simulink model "mrefrobotarm_modified_previous_y_previous_u_previous_ref"  (R2018b)
settings: Solver=FixedStepAuto  StartTime=0.0  StopTime=10  RelTol=1e-3  AbsTol=1e-6
undefined symbols (not defined in the file or in its folder): options, sfunxy2
libraries: neural x949, simulink x1
(part 16 of 31)

== system mrefrobotarm_modified_previous_y_previous_u_previous_ref/const_51_unstable/Layer 2/Delays 1 ==
  "p{2}" : Inport  PortDimensions=50
      mask Display: e = 0.06;c1 = [120 230 180]/255;c2 = ([120 230 180]+0)/(256+128);c3 = ([120 230 180]+128)/(256+128);patch([0 1 1 0],[0 0 1 1],c1);patch([0 1 1 1-e 1-e 0+e],[0 0 1 1-e 0+e 0+e],c2);patch([0 0 1 1-e 0+e 0+e],[0 1 1 1-e 1-e 0+e],c3);plot([0 1 1 0 0],[0 0 1 1 0]);
  mux : Mux  Inputs=1
      mask Display: e = 0.06;c1 = [120 150 230]/255;c2 = ([120 150 230]+0)/383;c3 = ([120 150 230]+128)/383;patch([0 1 1 0],[0 0 1 1],c1);patch([0 1 1 1-e 1-e 0+e],[0 0 1 1-e 0+e 0+e],c2);patch([0 0 1 1-e 0+e 0+e],[0 1 1 1-e 1-e 0+e],c3);plot([0 1 1 0 0],[0 0 1 1 0]);disp('Mux')
  "pd{2,1}" : Outport
      mask Display: e = 0.06;c1 = [120 230 180]/255;c2 = ([120 230 180]+0)/(256+128);c3 = ([120 230 180]+128)/(256+128);patch([0 1 1 0],[0 0 1 1],c1);patch([0 1 1 1-e 1-e 0+e],[0 0 1 1-e 0+e 0+e],c2);patch([0 0 1 1-e 0+e 0+e],[0 1 1 1-e 1-e 0+e],c3);plot([0 1 1 0 0],[0 0 1 1 0]);
  wires:
  "p{2}"/1 -> mux/1
  mux/1 -> "pd{2,1}"/1

== system mrefrobotarm_modified_previous_y_previous_u_previous_ref/const_51_unstable/Layer 2/LW{2,1} ==
  "ad{2,1}" : Inport  PortDimensions=50
      mask Display: e = 0.06;c1 = [120 230 180]/255;c2 = ([120 230 180]+0)/(256+128);c3 = ([120 230 180]+128)/(256+128);patch([0 1 1 0],[0 0 1 1],c1);patch([0 1 1 1-e 1-e 0+e],[0 0 1 1-e 0+e 0+e],c2);patch([0 0 1 1-e 0+e 0+e],[0 1 1 1-e 1-e 0+e],c3);plot([0 1 1 0 0],[0 0 1 1 0]);
  "IW{2,1}(1,:)'" : Constant  Value=[0.015906593054590668911973949661842198111116886138916015625;0.01820805169246907107005739590022130869328975677490234375;0.326514062945760741296652440723846666514873504638671875;-0.1966668405829790078342966808122582733631134033203125;0.50794780405529216249504997904296033084392547607421875;-1.7723192755342032089771464598015882074832916259765625;0.09304160139981214328042113947958569042384624481201171875;1.626950351079901491146983971702866256237030029296875;0.0493885885006573877031854635788477025926113128662109375;0.5968628191114031533714978650095872581005096435546875;0.09516382795030368935140785424664500169456005096435546875;-0.00046053148100815878562830363307512016035616397857666015625;0.228803574962702871431474704877473413944244384765625;0.01304940280174379275968110647454523132182657718658447265625;-0.0199995955487506961445465236693053157068789005279541015625;0.004623501465819892554398595763132107094861567020416259765625;-0.8655537125411705279276475266669876873493194580078125;0.1331348498208286823540902332752011716365814208984375;0.6018039174588725170877978598582558333873748779296875;-0.0483283123428327743287269413485773839056491851806640625;0.0179876365483312393445114452106281532905995845794677734375;0.0702157094976696705135310594414477236568927764892578125;0.0272840601000100164974515593030446325428783893585205078125;-0.0194226028672902784055764868753612972795963287353515625;0.01453041064602469088773428751437677419744431972503662109375;0.0020353394274947207709391960861466941423714160919189453125;0.21604466372356434522572499190573580563068389892578125;0.07193972134304969789919681488754577003419399261474609375;0.168790156870227914254201095900498330593109130859375;-0.04284208945847774174797706336903502233326435089111328125;0.0141586861150130617625908513446120196022093296051025390625;-0.0874432365739864214670973296961165033280849456787109375;1.09132254375588910733085867832414805889129638671875;0.08605488458340380952815706905312254093587398529052734375;0.46301273221957173209517577561200596392154693603515625;-0.09188314496760342786618735999581986106932163238525390625;0.0073916631840500179873032493560458533465862274169921875;-0.12453075105480236606236843499573296867311000823974609375;0.0473848129603824663735878175430116243660449981689453125;0.042029984239448529848015567722541163675487041473388671875;0.2885001240608235928419844640302471816539764404296875;0.0102703963665113119640981409474989050067961215972900390625;0.2209503318790606296584400070059928111732006072998046875;0.000582007111679681832239197092349058948457241058349609375;0.0706595064007065065680990301189012825489044189453125;0.031424509096391543827575532077389652840793132781982421875;0.062313879588255412234065744314648327417671680450439453125;0.5251181800068758231958554461016319692134857177734375;0.455409756693149481154847535435692407190799713134765625;0.0602594044245531590409115096917957998812198638916015625]
      mask Display: e = 0.06;c1 = [120 150 230]/255;c2 = ([120 150 230]+0)/383;c3 = ([120 150 230]+128)/383;patch([0 1 1 0],[0 0 1 1],c1);patch([0 1 1 1-e 1-e 0+e],[0 0 1 1-e 0+e 0+e],c2);patch([0 0 1 1-e 0+e 0+e],[0 1 1 1-e 1-e 0+e],c3);plot([0 1 1 0 0],[0 0 1 1 0]);disp('weights');
  Mux : Mux  Inputs=1
      mask Display: e = 0.06;c1 = [120 150 230]/255;c2 = ([120 150 230]+0)/383;c3 = ([120 150 230]+128)/383;patch([0 1 1 0],[0 0 1 1],c1);patch([0 1 1 1-e 1-e 0+e],[0 0 1 1-e 0+e 0+e],c2);patch([0 0 1 1-e 0+e 0+e],[0 1 1 1-e 1-e 0+e],c3);plot([0 1 1 0 0],[0 0 1 1 0]);disp('Mux');
  dotprod1 : neural/Weight Functions/dotprod
  "lz{2,1}" : Outport
      mask Display: e = 0.06;c1 = [120 230 180]/255;c2 = ([120 230 180]+0)/(256+128);c3 = ([120 230 180]+128)/(256+128);patch([0 1 1 0],[0 0 1 1],c1);patch([0 1 1 1-e 1-e 0+e],[0 0 1 1-e 0+e 0+e],c2);patch([0 0 1 1-e 0+e 0+e],[0 1 1 1-e 1-e 0+e],c3);plot([0 1 1 0 0],[0 0 1 1 0]);
  wires:
  "IW{2,1}(1,:)'"/1 -> dotprod1/1
  "ad{2,1}"/1 -> dotprod1/2
  dotprod1/1 -> Mux/1
  Mux/1 -> "lz{2,1}"/1

== system mrefrobotarm_modified_previous_y_previous_u_previous_ref/const_51traces_100/Layer 1/Delays 1 ==
  "p{1}" : Inport  PortDimensions=10
      mask Display: e = 0.06;c1 = [120 230 180]/255;c2 = ([120 230 180]+0)/(256+128);c3 = ([120 230 180]+128)/(256+128);patch([0 1 1 0],[0 0 1 1],c1);patch([0 1 1 1-e 1-e 0+e],[0 0 1 1-e 0+e 0+e],c2);patch([0 0 1 1-e 0+e 0+e],[0 1 1 1-e 1-e 0+e],c3);plot([0 1 1 0 0],[0 0 1 1 0]);
  mux : Mux  Inputs=1
      mask Display: e = 0.06;c1 = [120 150 230]/255;c2 = ([120 150 230]+0)/383;c3 = ([120 150 230]+128)/383;patch([0 1 1 0],[0 0 1 1],c1);patch([0 1 1 1-e 1-e 0+e],[0 0 1 1-e 0+e 0+e],c2);patch([0 0 1 1-e 0+e 0+e],[0 1 1 1-e 1-e 0+e],c3);plot([0 1 1 0 0],[0 0 1 1 0]);disp('Mux')
  "pd{1,1}" : Outport
      mask Display: e = 0.06;c1 = [120 230 180]/255;c2 = ([120 230 180]+0)/(256+128);c3 = ([120 230 180]+128)/(256+128);patch([0 1 1 0],[0 0 1 1],c1);patch([0 1 1 1-e 1-e 0+e],[0 0 1 1-e 0+e 0+e],c2);patch([0 0 1 1-e 0+e 0+e],[0 1 1 1-e 1-e 0+e],c3);plot([0 1 1 0 0],[0 0 1 1 0]);
  wires:
  "p{1}"/1 -> mux/1
  mux/1 -> "pd{1,1}"/1
